simulink model "dataflow"  (R2023b)
settings: Solver=VariableStepAuto  StartTime=0.0  StopTime=min_sample_time  RelTol=1e-3
values from neighbouring files (symbols this model uses):
  bit_samp = 12    [Copy_of_scatter_test.m]    (also in Zero_Crossing_Error.m; Zero_Crossing_Error_Optimized.m; fpga_script.m)
  f_ref = 10e6    (= 10000000)    [Copy_of_scatter_test.m]    (also in Zero_Crossing_Error.m; Zero_Crossing_Error_Optimized.m; fpga_script.m)
  f_samp = 60.94e6    (= 60940000)    [Copy_of_scatter_test.m]    (also in Zero_Crossing_Error.m; Zero_Crossing_Error_Optimized.m; fpga_script.m)
  f_sim = 160*f_samp    (= 9750400000)    [Copy_of_scatter_test.m]    (also in Zero_Crossing_Error.m; fpga_script.m)
  test_gain = 1/10    (= 0.1)    [Copy_of_scatter_test.m]    (also in Zero_Crossing_Error.m; fpga_script.m)
  test_phase = test_phase_deg/180*pi    [Copy_of_scatter_test.m]    (also in Zero_Crossing_Error.m; fpga_script.m = 0.191986217719)
libraries: simulink_extras x2, dspsigops x1
settings Model: Creator=matej  LastModifiedBy=matej

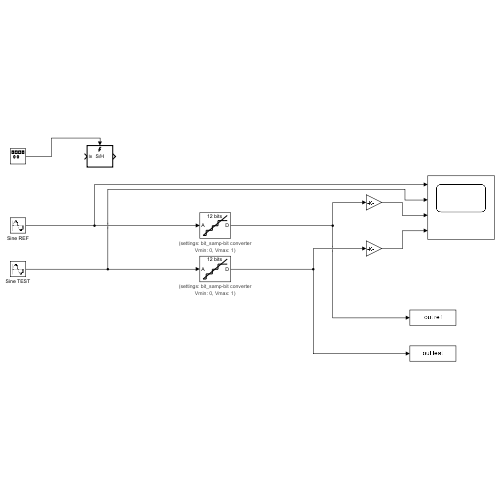
[thumbnail: Simulink's stored preview of the top-level diagram]
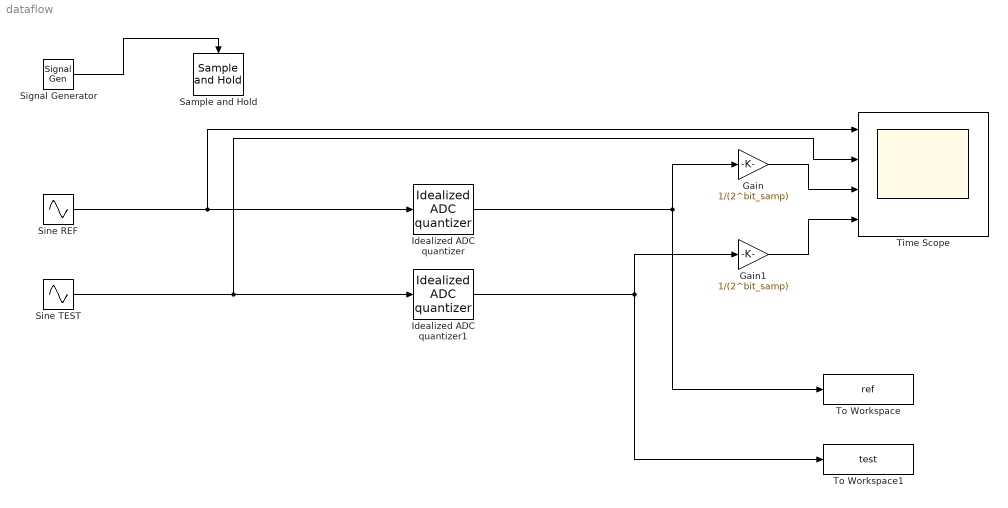
== system dataflow ==
  Gain : Gain  Gain=1/(2^bit_samp)
  Gain1 : Gain  Gain=1/(2^bit_samp)
  Idealized ADC quantizer : simulink_extras/Additional Discrete/Idealized ADC quantizer  NumberOfConverterBits=bit_samp  Vmin=0  Vmax=1  OutputDataType=int16  OutputNegativeValues=off
  Idealized ADC quantizer1 : simulink_extras/Additional Discrete/Idealized ADC quantizer  NumberOfConverterBits=bit_samp  Vmin=0  Vmax=1  OutputDataType=int16  OutputNegativeValues=off
  Sample and Hold : dspsigops/Sample and Hold  trig=Rising edge  initCond=0  latchinput=off
  Signal Generator : SignalGenerator  WaveForm=square  Frequency=f_samp
  Sine REF : Sin  Amplitude=1/2  Bias=1/2  Frequency=2*pi*f_ref  SampleTime=1/f_sim
  Sine TEST : Sin  Amplitude=1/2*test_gain  Bias=1/2  Frequency=2*pi*f_ref  Phase=test_phase  SampleTime=1/f_sim
  Time Scope : Scope  NumInputPorts=4
  To Workspace : ToWorkspace  VariableName=ref  SampleTime=1/f_samp
      settings: Save2DSignal=2-D array (concatenate along first dimension)
  To Workspace1 : ToWorkspace  VariableName=test  SampleTime=1/f_samp
      settings: Save2DSignal=2-D array (concatenate along first dimension)
  wires:
  Idealized ADC quantizer/1 -> Gain/1, To Workspace/1
  Idealized ADC quantizer1/1 -> To Workspace1/1, Gain1/1
  Sine REF/1 -> Idealized ADC quantizer/1, Time Scope/1
  Sine TEST/1 -> Idealized ADC quantizer1/1, Time Scope/2
  Gain/1 -> Time Scope/3
  Gain1/1 -> Time Scope/4
  Signal Generator/1 -> Sample and Hold/Trigger
